simulink model "escooter_sequence_diagram_overheating"  (R2025b)
settings: Solver=VariableStepAuto  StartTime=0.0  StopTime=10.0  RelTol=1e-3
settings Model: Creator=320236370  LastModifiedBy=320236370

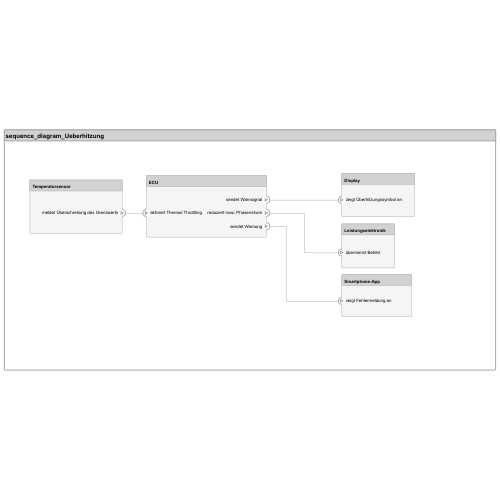
[thumbnail: Simulink's stored preview of the top-level diagram]
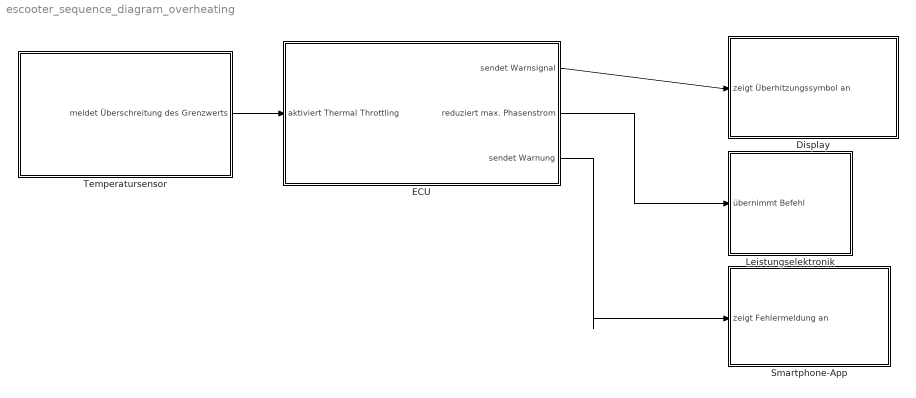
== system escooter_sequence_diagram_overheating ==
  Display : Subsystem
      settings: PortSchema="{\"entries\":[{\"content\":{\"headerSize\":26,\"margin\":15,\"minimumSpacing\":25,\"sides\":[{\"content\":{\"connectorIds\":[\"In1\"]},\"type\":\"ConnectorPlacement.EquallySpacedRectSide\",\"uuid\":\"3d49029f-ff69-43f0-9083-eb7baed04898\"},{\"content\":{\"side\":\"RIGHT\"},\"type\":\"ConnectorPlacement.EquallySpacedRectSide\",\"uuid\":\"1597d90c-c332-40d9-8a70-68f04d256300\"},{\"content\":{\"side\":\"TOP\"},\"type\":\"ConnectorPlacement.EquallySpacedRectSide\",\"uuid\":\"ad895052-9fa6-4dfa-a28f-1843b80a8a3f\"}]},\"type\":\"ConnectorPlacement.EquallySpacedConnector\",\"uuid\":\"8d35fef0-5689-4d8b-850c-97501fa910c2\"}],\"packageUris\":[\"http://schema.mathworks.com/mf0/Connector/R2020b\"],\"version\":\"1.0\"}"
  ECU : Subsystem
      settings: PortSchema="{\"entries\":[{\"content\":{\"headerSize\":26,\"margin\":15,\"minimumSpacing\":25,\"sides\":[{\"content\":{\"connectorIds\":[\"In1\"]},\"type\":\"ConnectorPlacement.EquallySpacedRectSide\",\"uuid\":\"3d49029f-ff69-43f0-9083-eb7baed04898\"},{\"content\":{\"connectorIds\":[\"Out1\",\"Out2\",\"Out3\"],\"side\":\"RIGHT\"},\"type\":\"ConnectorPlacement.EquallySpacedRectSide\",\"uuid\":\"1597d90c-c332-40d9-8a70-68f04d256300\"},{\"content\":{\"side\":\"TOP\"},\"type\":\"ConnectorPlacement.EquallySpacedRectSide\",\"uuid\":\"ad895052-9fa6-4dfa-a28f-1843b80a8a3f\"}]},\"type\":\"ConnectorPlacement.EquallySpacedConnector\",\"uuid\":\"8d35fef0-5689-4d8b-850c-97501fa910c2\"}],\"packageUris\":[\"http://schema.mathworks.com/mf0/Connector/R2020b\"],\"version\":\"1.0\"}"
  Leistungselektronik : Subsystem
      settings: PortSchema="{\"entries\":[{\"content\":{\"headerSize\":26,\"margin\":15,\"minimumSpacing\":25,\"sides\":[{\"content\":{\"connectorIds\":[\"In1\"]},\"type\":\"ConnectorPlacement.EquallySpacedRectSide\",\"uuid\":\"3d49029f-ff69-43f0-9083-eb7baed04898\"},{\"content\":{\"side\":\"RIGHT\"},\"type\":\"ConnectorPlacement.EquallySpacedRectSide\",\"uuid\":\"1597d90c-c332-40d9-8a70-68f04d256300\"},{\"content\":{\"side\":\"TOP\"},\"type\":\"ConnectorPlacement.EquallySpacedRectSide\",\"uuid\":\"ad895052-9fa6-4dfa-a28f-1843b80a8a3f\"}]},\"type\":\"ConnectorPlacement.EquallySpacedConnector\",\"uuid\":\"8d35fef0-5689-4d8b-850c-97501fa910c2\"}],\"packageUris\":[\"http://schema.mathworks.com/mf0/Connector/R2020b\"],\"version\":\"1.0\"}"
  Smartphone-App : Subsystem
      settings: PortSchema="{\"entries\":[{\"content\":{\"headerSize\":26,\"margin\":15,\"minimumSpacing\":25,\"sides\":[{\"content\":{\"connectorIds\":[\"In1\"]},\"type\":\"ConnectorPlacement.EquallySpacedRectSide\",\"uuid\":\"3d49029f-ff69-43f0-9083-eb7baed04898\"},{\"content\":{\"side\":\"RIGHT\"},\"type\":\"ConnectorPlacement.EquallySpacedRectSide\",\"uuid\":\"1597d90c-c332-40d9-8a70-68f04d256300\"},{\"content\":{\"side\":\"TOP\"},\"type\":\"ConnectorPlacement.EquallySpacedRectSide\",\"uuid\":\"ad895052-9fa6-4dfa-a28f-1843b80a8a3f\"}]},\"type\":\"ConnectorPlacement.EquallySpacedConnector\",\"uuid\":\"8d35fef0-5689-4d8b-850c-97501fa910c2\"}],\"packageUris\":[\"http://schema.mathworks.com/mf0/Connector/R2020b\"],\"version\":\"1.0\"}"
  Temperatursensor : Subsystem
      settings: PortSchema="{\"entries\":[{\"content\":{\"headerSize\":26,\"margin\":15,\"minimumSpacing\":25,\"sides\":[{\"content\":{},\"type\":\"ConnectorPlacement.EquallySpacedRectSide\",\"uuid\":\"3d49029f-ff69-43f0-9083-eb7baed04898\"},{\"content\":{\"connectorIds\":[\"Out1\"],\"side\":\"RIGHT\"},\"type\":\"ConnectorPlacement.EquallySpacedRectSide\",\"uuid\":\"1597d90c-c332-40d9-8a70-68f04d256300\"},{\"content\":{\"side\":\"TOP\"},\"type\":\"ConnectorPlacement.EquallySpacedRectSide\",\"uuid\":\"ad895052-9fa6-4dfa-a28f-1843b80a8a3f\"}]},\"type\":\"ConnectorPlacement.EquallySpacedConnector\",\"uuid\":\"8d35fef0-5689-4d8b-850c-97501fa910c2\"}],\"packageUris\":[\"http://schema.mathworks.com/mf0/Connector/R2020b\"],\"version\":\"1.0\"}"
  wires:
  Temperatursensor/1(meldet Überschreitung des Grenzwerts) -> ECU/1(aktiviert Thermal Throttling)
  ECU/1(sendet Warnsignal) -> Display/1(zeigt Überhitzungssymbol an)
  ECU/2(reduziert max. Phasenstrom) -> Leistungselektronik/1(übernimmt Befehl)
  ECU/3(sendet Warnung) -> Smartphone-App/1(zeigt Fehlermeldung an)

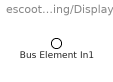
== system escooter_sequence_diagram_overheating/Display ==
  Bus Element In1 : Inport  PortName=zeigt Überhitzungssymbol an

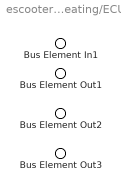
== system escooter_sequence_diagram_overheating/ECU ==
  Bus Element In1 : Inport  PortName=aktiviert Thermal Throttling
  Bus Element Out1 : Outport  PortName=sendet Warnsignal
  Bus Element Out2 : Outport  Port=2  PortName=reduziert max. Phasenstrom
  Bus Element Out3 : Outport  Port=3  PortName=sendet Warnung

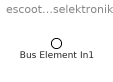
== system escooter_sequence_diagram_overheating/Leistungselektronik ==
  Bus Element In1 : Inport  PortName=übernimmt Befehl

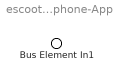
== system escooter_sequence_diagram_overheating/Smartphone-App ==
  Bus Element In1 : Inport  PortName=zeigt Fehlermeldung an

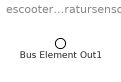
== system escooter_sequence_diagram_overheating/Temperatursensor ==
  Bus Element Out1 : Outport  PortName=meldet Überschreitung des Grenzwerts
